simulink model "gm_sampleModel1677_5_sub_sub"  (R2023a)
settings: Solver=VariableStepAuto  StartTime=0.0  StopTime=10.0  RelTol=1e-3
libraries: hdlsllib x4, simulink x3
settings Model: Creator=user1  LastModifiedBy=user1
settings OptimizationCC: BlockReduction=off  ConditionallyExecuteInputs=off
settings DebuggingCC: InheritedTsInSrcMsg=none

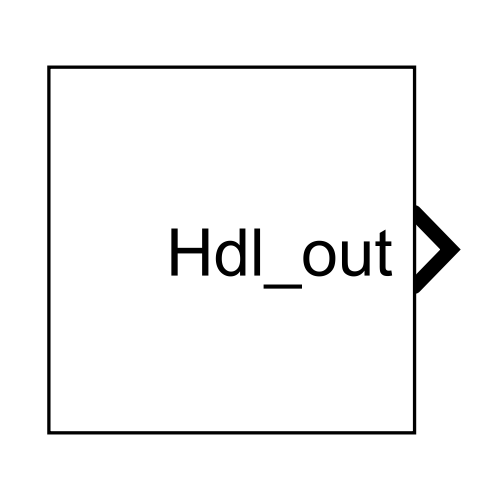
[thumbnail: Simulink's stored preview of the top-level diagram]
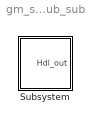
== system gm_sampleModel1677_5_sub_sub ==
  Subsystem : Subsystem

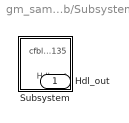
== system gm_sampleModel1677_5_sub_sub/Subsystem ==
  Subsystem : Subsystem
  Hdl_out : Outport  OutDataTypeStr=uint8

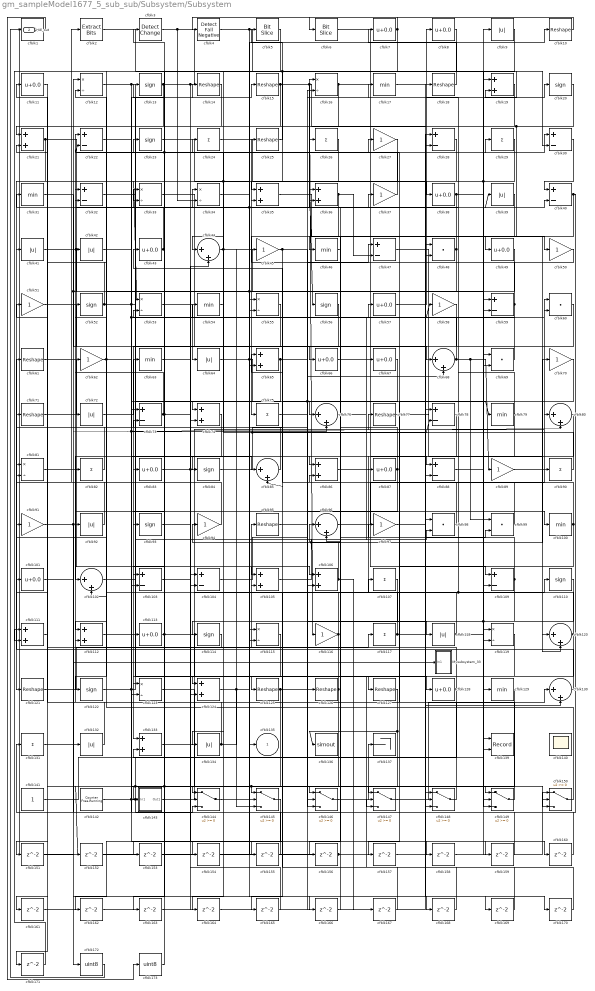
== system gm_sampleModel1677_5_sub_sub/Subsystem/Subsystem ==
  Mysubsystem_33 : Subsystem  TreatAsAtomicUnit=on  RTWFcnName=Mysubsystem_33
      settings: RTWFcnNameOpts=User specified  RTWFileNameOpts=Use function name
  cfblk1 : simulink/Logic and Bit Operations/Bit Set  iBit=0
      settings: LibrarySourceBlock=|
      | hdlsllib/Logic and Bit
      | Operations/Bit Set
  cfblk{10,14..15,18,25,61,71,77,95,121,125..127} (13 alike) : Reshape
  cfblk{17,31,46,54,63,79,100,129} (8 alike) : MinMax  OutDataTypeStr=uint8
  cfblk{7..8,11,38,43,49,57,66..67,83,87,101,113,128} (14 alike) : Bias  Bias=0.0  SaturateOnIntegerOverflow=off
  cfblk{44,68,76,80,85,96,102,120,130} (9 alike) : Sum  Inputs=|++  OutDataTypeStr=uint8
  cfblk{22,28,30,32,40,47,59,73,78,88,103..104,109} (13 alike) : Sum  Inputs=+-  OutDataTypeStr=uint8
  cfblk{19,21,35..36,65,74,86,105..106,111..112,124,133} (13 alike) : Sum  OutDataTypeStr=uint8
  cfblk{24,26,29,75,82,90,107,117,131} (9 alike) : Sum  Inputs=+  OutDataTypeStr=uint8
  cfblk{13,20,23,52,56,84,93,110,114,122} (10 alike) : Signum
  cfblk{12,16,33..34,53,55,81,115,119,123} (10 alike) : Product  Inputs=*/  OutDataTypeStr=uint8  RndMeth=Zero  SaturateOnIntegerOverflow=on
  cfblk{27,37,45,50..51,58,62,70,89,91,94,97,116} (13 alike) : Gain  OutDataTypeStr=uint8
  cfblk{9,39,41..42,64,72,92,118,132,134} (10 alike) : Abs  OutDataTypeStr=uint8  SaturateOnIntegerOverflow=off
  cfblk136 : ToWorkspace  VariableName=simout  SaveFormat=Timeseries  SampleTime=-1
  cfblk137 : Terminator
  cfblk139 : Record  FileSettingsInternal="{\"entries\":[{\"content\":{\"excelSettings\":{\"content\":{},\"type\":\"Streamout.ExcelSettings\"}},\"type\":\"Streamout.FileSettingStorage\",\"uuid\":\"\"}],\"packageUris\":[\"http:\\/\\/schema.mathworks.com\\/mf0\\/streamout_blocks\\/R2020a\"],\"version\":\"1.0\"}"  Layout=[1 1]  SignalsInternal="{\"entries\":[{\"content\":{\"signals\":[{\"content\":{\"blockPath\":[],\"dimensions\":[1],\"domain\":\"\",\"lineColor\":\"#a2142f\",\"plots\":[1],\"port\":1,\"signalID\":25839,\"signalName\":\"cfblk4\"},\"type\":\"RecordBlkView.Signal\",\"uuid\":\"\"},{\"content\":{\"blockPath\":[],\"dimensions\":[1],\"domain\":\"\",\"lineColor\":\"#139fff\",\"plots\":[1],\"port\":2,\"signalID\":25842,\"signalName\":\"cfblk109\"},\"type\":\"RecordBlkView.Signal\",\"uuid\":\"\"}]},\"type\":\"RecordBlkView.InputSignals\",\"uuid\":\"\"}],\"packageUris\":[\"http:\\/\\/schema.mathworks.com\\/mf0\\/streamout_blocks\\/R2020a\"],\"version\":\"1.0\"}"  VisualizationBindings="{\"xyplotplugin\":{\"info\":[{\"series\":[{\"bindingParametersList\":[{\"parameter\":\"X-Axis\",\"signalID\":25839,\"signalName\":\"cfblk4\"},{\"parameter\":\"Y-Axis\",\"signalID\":25842,\"signalName\":\"cfblk109\"}],\"seriesID\":34496}],\"subplotID\":1}]}}"  CompatibilityTag=XY  st=-1
  cfblk140 : Scope
      settings: Floating=on
  cfblk141 : Constant  OutDataTypeStr=uint8  SampleTime=-1
  cfblk142 : hdlsllib/Sources/Counter Free-Running  NumBits=16  tsamp=-1
  cfblk143 : Subsystem
      settings: LibrarySourceBlock=|
      | hdlsllib/Ports &
      | Subsystems/Subsystem
  cfblk{144..150} (7 alike) : Switch  OutDataTypeStr=uint8  SaturateOnIntegerOverflow=off  InputSameDT=off
  cfblk{151..171} (21 alike) : Delay  SampleTime=1
  cfblk172 : DataTypeConversion  OutDataTypeStr=uint8  SaturateOnIntegerOverflow=off  RndMeth=Floor
  cfblk173 : DataTypeConversion  OutDataTypeStr=uint8  SaturateOnIntegerOverflow=off  RndMeth=Floor
  cfblk2 : simulink/Logic and Bit Operations/Extract Bits  bitsToExtract=Upper half  numBits=8  bitIdxRange=[0 7]  outScalingMode=Preserve fixed-point scaling
      settings: LibrarySourceBlock=|
      | hdlsllib/Logic and Bit
      | Operations/Extract Bits
  cfblk3 : simulink/Logic and Bit Operations/Detect Change  vinit=0  OutDataTypeStr=uint8
      settings: LibrarySourceBlock=|
      | hdlsllib/Logic and Bit
      | Operations/Detect
      | Change
  cfblk4 : hdlsllib/Logic and Bit Operations/Detect Fall Negative  vinit=0  OutDataTypeStr=uint8
  cfblk{48,60,69,98..99} (5 alike) : DotProduct  OutDataTypeStr=uint8
  cfblk5 : hdlsllib/Logic and Bit Operations/Bit Slice  lidx=7  ridx=0
  cfblk6 : hdlsllib/Logic and Bit Operations/Bit Slice  lidx=7  ridx=0
  cfblk135 : Outport  OutDataTypeStr=uint8  VectorParamsAs1DForOutWhenUnconnected=off
  Hdl_out : Outport  Port=2  OutDataTypeStr=uint8
  wires:
  cfblk12/1 -> cfblk100/1, cfblk127/1
  cfblk20/1 -> cfblk49/1, cfblk116/1
  cfblk16/1 -> cfblk21/1, cfblk109/1
  cfblk21/1 -> cfblk28/2, cfblk121/1
  cfblk86/1 -> cfblk110/1
  cfblk58/1 -> cfblk133/1
  cfblk116/1 -> cfblk72/1, cfblk95/1
  cfblk29/1 -> cfblk69/2, cfblk56/1
  cfblk118/1 -> cfblk81/2, cfblk19/1
  cfblk85/1 -> cfblk22/1
  cfblk66/1 -> cfblk88/1
  cfblk92/1 -> cfblk2/1
  cfblk32/1 -> cfblk76/1
  cfblk130/1 -> cfblk61/1
  cfblk128/1 -> cfblk101/1, cfblk133/2
  cfblk47/1 -> cfblk129/1
  cfblk68/1 -> cfblk24/1, cfblk99/1, cfblk89/1
  cfblk102/1 -> cfblk15/1
  cfblk117/1 -> cfblk99/2, cfblk91/1
  cfblk104/1 -> cfblk29/1
  cfblk71/1 -> cfblk23/1
  cfblk30/1 -> cfblk40/1
  cfblk13/1 -> cfblk102/2, cfblk149/3, cfblk19/2
  cfblk38/1 -> cfblk35/2, cfblk9/1
  cfblk72/1 -> cfblk63/1
  cfblk40/1 -> cfblk86/1, cfblk131/1
  cfblk143/1(Out1) -> cfblk107/1
  cfblk89/1 -> cfblk60/1
  cfblk4/1 -> cfblk150/3, cfblk139/1
  cfblk148/1 -> cfblk57/1
  cfblk6/1 -> cfblk50/1
  cfblk48/1 -> cfblk37/1, cfblk103/2, cfblk145/2
  cfblk83/1 -> cfblk106/1, cfblk77/1
  cfblk53/1 -> cfblk64/1
  cfblk134/1 -> cfblk45/1, cfblk32/1
  cfblk133/1 -> cfblk80/1
  cfblk76/1 -> cfblk60/2
  cfblk77/1 -> cfblk120/1
  cfblk63/1 -> cfblk68/1
  cfblk22/1 -> cfblk105/1
  cfblk122/1 -> cfblk146/2, cfblk98/2
  cfblk147/1 -> cfblk130/1
  cfblk146/1 -> cfblk137/1
  cfblk94/1 -> cfblk51/1
  cfblk106/1 -> cfblk167/1, cfblk94/1
  cfblk57/1 -> cfblk8/1
  cfblk69/1 -> cfblk27/1
  cfblk121/1 -> cfblk117/1
  cfblk100/1 -> cfblk43/1, cfblk147/1
  cfblk39/1 -> cfblk75/1
  cfblk120/1 -> cfblk147/3, cfblk97/1, cfblk18/1
  cfblk44/1 -> cfblk146/3, cfblk124/1
  cfblk41/1 -> cfblk88/2, cfblk16/1
  cfblk99/1 -> cfblk71/1
  cfblk33/1 -> cfblk115/1
  cfblk127/1 -> cfblk136/1, cfblk153/1, cfblk152/1
  cfblk87/1 -> cfblk106/2, cfblk34/1
  cfblk18/1 -> cfblk7/1
  cfblk36/1 -> cfblk47/2, cfblk46/1
  cfblk51/1 -> cfblk66/1
  cfblk126/1 -> cfblk155/1, cfblk52/1
  cfblk123/1 -> cfblk149/1
  cfblk142/1 -> cfblk113/1, cfblk144/3, cfblk148/2, cfblk119/2
  cfblk45/1 -> cfblk85/2, cfblk118/1
  cfblk74/1 -> cfblk102/1
  cfblk19/1 -> cfblk36/1
  cfblk95/1 -> cfblk68/2
  cfblk81/1 -> cfblk124/2
  cfblk60/1 -> cfblk125/1
  cfblk79/1 -> cfblk33/1, cfblk92/1
  cfblk24/1 -> cfblk38/1
  cfblk88/1 -> cfblk40/2
  cfblk73/1 -> cfblk42/1, cfblk158/1, cfblk93/1
  cfblk82/1 -> cfblk32/2
  cfblk129/1 -> cfblk163/1, cfblk145/1
  cfblk115/1 -> cfblk123/1
  cfblk5/1 -> cfblk44/1
  cfblk31/1 -> cfblk65/2, cfblk59/2
  cfblk105/1 -> cfblk70/1, cfblk67/1
  cfblk84/1 -> cfblk78/2, cfblk17/1
  cfblk35/1 -> cfblk120/2
  cfblk43/1 -> cfblk11/1, cfblk103/1
  cfblk101/1 -> cfblk132/1
  cfblk28/1 -> cfblk164/1, cfblk53/1
  cfblk75/1 -> cfblk20/1, cfblk79/1
  cfblk119/1 -> cfblk134/1
  cfblk98/1 -> cfblk65/1
  cfblk62/1 -> cfblk12/2, cfblk14/1
  cfblk49/1 -> cfblk112/1
  cfblk61/1 -> cfblk104/2
  cfblk97/1 -> cfblk130/2
  cfblk15/1 -> cfblk114/1, cfblk148/1, cfblk26/1
  cfblk42/1 -> cfblk160/1, cfblk76/2
  cfblk26/1 -> cfblk41/1
  cfblk112/1 -> cfblk58/1, cfblk30/1
  cfblk149/1 -> cfblk73/2
  cfblk52/1 -> cfblk21/2, cfblk85/1, cfblk78/1
  cfblk96/1 -> cfblk90/1
  cfblk124/1 -> cfblk145/3, cfblk39/1, cfblk10/1
  cfblk3/1 -> cfblk34/2, cfblk55/1
  cfblk111/1 -> cfblk31/1
  cfblk10/1 -> cfblk6/1
  cfblk70/1 -> cfblk87/1
  cfblk91/1 -> cfblk80/2, Mysubsystem_33/1(In1)
  cfblk90/1 -> cfblk54/1
  cfblk59/1 -> cfblk53/2, cfblk25/1
  cfblk8/1 -> cfblk111/2
  cfblk110/1 -> cfblk144/1
  cfblk109/1 -> cfblk86/2, cfblk148/3, cfblk139/2
  cfblk64/1 -> cfblk146/1, cfblk149/2
  cfblk114/1 -> cfblk112/2
  cfblk50/1 -> cfblk48/2
  cfblk2/1 -> cfblk30/2
  cfblk150/1 -> cfblk62/1
  cfblk9/1 -> cfblk143/1(In1), cfblk35/1
  cfblk132/1 -> cfblk81/1
  cfblk25/1 -> cfblk5/1
  cfblk55/1 -> cfblk83/1
  cfblk46/1 -> cfblk96/2
  cfblk103/1 -> cfblk144/2
  cfblk7/1 -> cfblk82/1, cfblk4/1
  cfblk107/1 -> cfblk115/2
  cfblk65/1 -> cfblk123/2, cfblk126/1
  cfblk141/1 -> cfblk119/1
  cfblk113/1 -> cfblk33/2, cfblk128/1
  cfblk125/1 -> cfblk161/1, cfblk47/1
  cfblk27/1 -> cfblk84/1, cfblk122/1
  cfblk37/1 -> cfblk22/2, cfblk3/1
  cfblk23/1 -> cfblk135/1
  cfblk54/1 -> cfblk74/1
  cfblk14/1 -> cfblk151/1
  cfblk152/1 -> cfblk150/2
  cfblk153/1 -> cfblk55/2
  cfblk56/1 -> cfblk154/1
  cfblk154/1 -> cfblk150/1
  cfblk155/1 -> cfblk12/1
  cfblk78/1 -> cfblk156/1
  cfblk156/1 -> Hdl_out/1, cfblk109/2
  cfblk80/1 -> cfblk157/1
  cfblk157/1 -> cfblk59/1
  cfblk158/1 -> cfblk69/1
  cfblk93/1 -> cfblk159/1
  cfblk159/1 -> cfblk96/1
  cfblk160/1 -> cfblk73/1
  cfblk161/1 -> cfblk28/1
  cfblk145/1 -> cfblk162/1
  cfblk162/1 -> cfblk44/2
  cfblk163/1 -> cfblk74/2
  cfblk164/1 -> cfblk16/2
  cfblk67/1 -> cfblk165/1
  cfblk165/1 -> cfblk104/1
  cfblk34/1 -> cfblk166/1
  cfblk166/1 -> cfblk36/2
  cfblk167/1 -> cfblk105/2
  cfblk131/1 -> cfblk168/1
  cfblk168/1 -> cfblk147/2
  cfblk144/1 -> cfblk169/1
  cfblk169/1 -> cfblk98/1
  cfblk17/1 -> cfblk170/1
  cfblk170/1 -> cfblk48/1
  cfblk11/1 -> cfblk171/1
  cfblk171/1 -> cfblk111/1
  cfblk151/1 -> cfblk172/1
  cfblk172/1 -> cfblk1/1
  cfblk1/1 -> cfblk173/1
  cfblk173/1 -> cfblk13/1

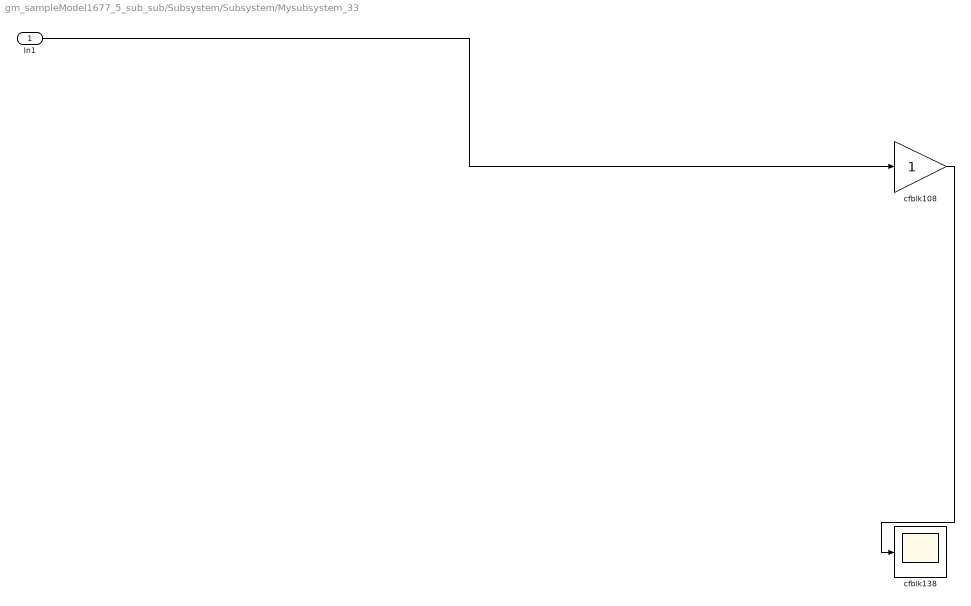
== system gm_sampleModel1677_5_sub_sub/Subsystem/Subsystem/Mysubsystem_33 ==
  In1 : Inport
  cfblk108 : Gain
  cfblk138 : Scope
  wires:
  In1/1 -> cfblk108/1
  cfblk108/1 -> cfblk138/1

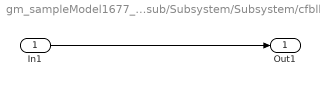
== system gm_sampleModel1677_5_sub_sub/Subsystem/Subsystem/cfblk143 ==
  In1 : Inport
  Out1 : Outport
  wires:
  In1/1 -> Out1/1
